simulink model "Flux_Nonsensor_pmsm"  (R2024a)
settings: Solver=FixedStepDiscrete  StartTime=0.0  StopTime=2  FixedStep=Fixed_Step_Size  RelTol=1e-3
InitFcn:
  | Flux_Nonsensor_data_new
values from neighbouring files (symbols this model uses):
  A = 1    [saddleToDuty.m]
  BandwidthCurrentPI = 1256*1.5    (= 1884)    [Flux_Nonsensor_data_new.m]
  Fixed_Step_Size = 1e-6    (= 1e-06)    [Flux_Nonsensor_data_new.m]
  Flux = 0.01837    [Flux_Nonsensor_data_new.m]
  Gamma = mpt.Parameter    [Flux_Nonsensor_data_new.m]
  Ld = 0.0001    [Flux_Nonsensor_data_new.m]
  Lq = 0.0001040    (= 0.000104)    [Flux_Nonsensor_data_new.m]
  Ls = 0.000195185    [Flux_Nonsensor_data_new.m]
  MaxVoltage = 10    [Flux_Nonsensor_data_new.m]
  pll_omega = mpt.Parameter    [Flux_Nonsensor_data_new.m]
  pll_xi = mpt.Parameter    [Flux_Nonsensor_data_new.m]
  PolePairs = 3    [Flux_Nonsensor_data_new.m]
  Rs = 0.02065    [Flux_Nonsensor_data_new.m]
  Speed_Ki = mpt.Parameter    [Flux_Nonsensor_data_new.m]
  Speed_Kp = mpt.Parameter    [Flux_Nonsensor_data_new.m]
  Speed_PI_OutputMax = 8    [Flux_Nonsensor_data_new.m]
  Speed_PI_OutputMin = -8    [Flux_Nonsensor_data_new.m]
  TsBSP = 1e-4    (= 0.0001)    [Flux_Nonsensor_data_new.m]
  TsBSP_MODEL = 2.5e-5    (= 2.5e-05)    [Flux_Nonsensor_data_new.m]
  TsFOC = 1e-4    (= 0.0001)    [Flux_Nonsensor_data_new.m]
undefined symbols (not defined in the file or in its folder): DiscIntNeverNeededParam, magnitude
libraries: slpidlib x3, mcbplantlib x1, spsDCVoltageSourceLib x1, spsGroundLib x1, autolibpmsminterior x1, spsPermanentMagnetSynchronousMachineLib x1, simulink x1, spsThreePhaseVIMeasurementLib x1, spsUniversalBridgeLib x1, sps_lib x1
settings Model: Creator=Administrator  LastModifiedBy=wanjietian
settings SolverCC: AlgebraicLoopSolver=TrustRegion
settings OptimizationCC: DefaultParameterBehavior=Inlined  UseDivisionForNetSlopeComputation=on  GainParamInheritBuiltInType=on  UseFloatMulNetSlope=on  InlineInvariantSignals=on  PassReuseOutputArgsAs=Individual arguments  ZeroExternalMemoryAtStartup=off  ZeroInternalMemoryAtStartup=off  NoFixptDivByZeroProtection=on  EfficientFloat2IntCast=on  LifeSpan=1  OptimizeBlockOrder=speed  DifferentSizesBufferReuse=on  EfficientTunableParamExpr=on
settings DebuggingCC: ParameterPrecisionLossMsg=none  ParameterTunabilityLossMsg=error  UnconnectedInputMsg=warning  UnconnectedOutputMsg=warning  UnconnectedLineMsg=warning
settings HardwareCC: ProdBitPerPointer=32  ProdBitPerSizeT=32  ProdBitPerPtrDiffT=32  ProdLargestAtomicInteger=Long  ProdLargestAtomicFloat=Double  ProdWordSize=32  ProdLongLongMode=on  ProdHWDeviceType=NXP->Cortex-M4
settings ModelReferenceCC: EnableRefExpFcnMdlSchedulingChecks=on  ModelReferenceNumInstancesAllowed=Single
settings SFSimCC: MATLABDynamicMemAlloc=off
settings RTWCC: Description=Embedded Coder  SystemTargetFile=ert.tlc  GenCodeOnly=on  TemplateMakefile=ert_default_tmf  GenerateReport=on  BuildConfiguration=Faster Runs  LaunchReport=on  GPUComputeCapability=3.5  DLArmComputeVersion=19.05
settings CodeAppCC: ForceParamTrailComments=on  IgnoreCustomStorageClasses=off  MaxIdLength=64  OperatorAnnotations=on  SimulinkDataObjDesc=on  SFDataObjDesc=on  CustomSymbolStrGlobalVar=rt$N$M  CustomSymbolStrType=$N$M  CustomSymbolStrFcn=$N$M$F  CustomSymbolStrMacro=$N$M  InsertBlockDesc=on
settings ERTTargetCC: TargetLangStandard=C99 (ISO)  GenerateSampleERTMain=on  IncludeMdlTerminateFcn=off  CombineSignalStateStructs=on  IncludeFileDelimiter=UseQuote  SupportAbsoluteTime=off  SupportComplex=off  SupportNonInlinedSFcns=on  InlinedParameterPlacement=NonHierarchical  ERTCustomFileTemplate=example_file_process.tlc  GlobalDataDefinition=InSeparateSourceFile  DataDefinitionFile=global_mcu_adc_isr.c  GlobalDataReference=InSeparateHeaderFile  DataReferenceFile=global_mcu_adc_isr.h

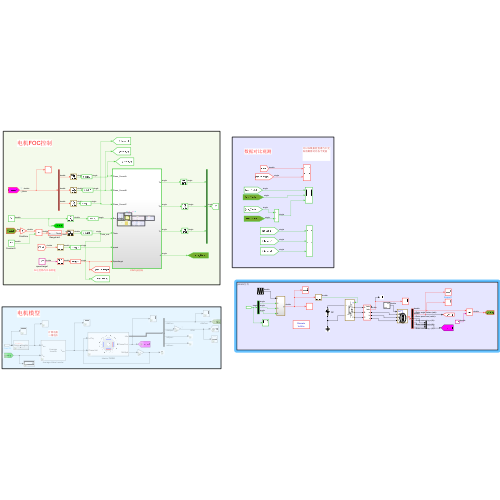
[thumbnail: Simulink's stored preview of the top-level diagram]
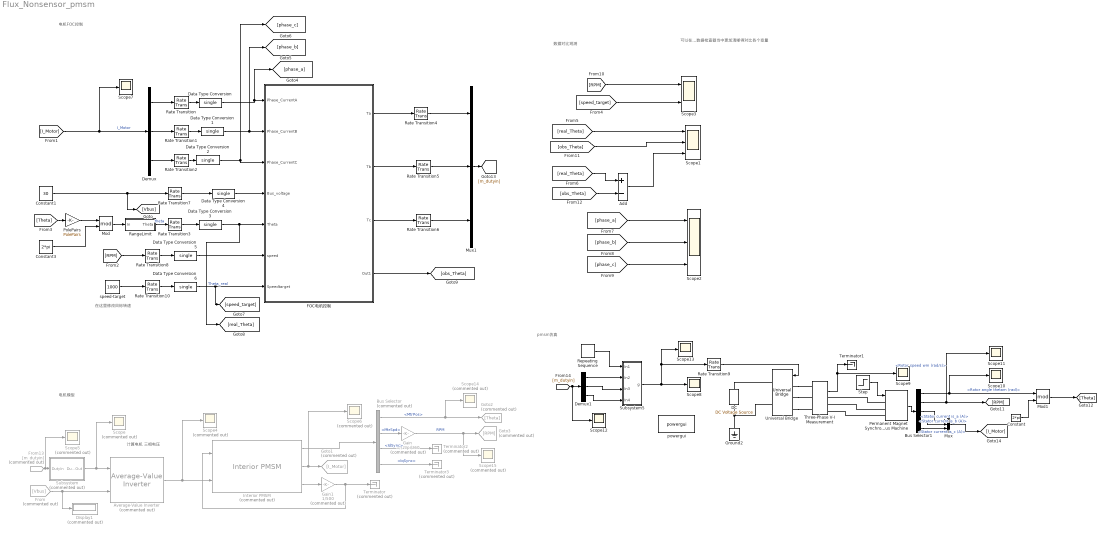
== system Flux_Nonsensor_pmsm ==
  note: pmsm仿真
  note: 可以在数据检查器当中更加清晰得对比各个变量
  note: 数据对比观测
  note: 计算电机
      | 三相电压
  note: 在这里修改目标转速
  note: 电机FOC控制
  note: 电机模型
  Add : Sum  Inputs=+-  OutDataTypeStr=single
  Average-Value Inverter : mcbplantlib/Average-Value Inverter  Commented=on
  Bus Selector : BusSelector  Commented=on  OutputSignals=MtrPos,MtrSpd,IdSync,IqSync
  Bus Selector1 : BusSelector  OutputSignals=Rotor angle thetam (rad),Rotor speed wm (rad/s),Stator current is_a (A),Stator current is_b (A),Stator current is_c (A)
  Constant : Constant  Value=2*pi
  Constant1 : Constant  Value=30  SampleTime=TsBSP
  "Constant3  " : Constant  Value=2*pi  SampleTime=TsBSP
  "DC " : spsDCVoltageSourceLib/DC Voltage Source  Amplitude=24  Measurements=Voltage
  Data Type Conversion{,1..6} (7 alike) : DataTypeConversion  OutDataTypeStr=single  SaturateOnIntegerOverflow=off  RndMeth=Floor
  Demux : Demux  Outputs=3
  Demux1 : Demux  Outputs=3
  Display1 : Display  Commented=on
  FOC电机控制 : Subsystem  TreatAsAtomicUnit=on  SystemSampleTime=TsFOC
  From : From  Commented=on  GotoTag=Vbus
  From13 : From  Commented=on  GotoTag=m_dutyin
  Gain : Gain  Commented=on  Gain=1/(2*pi)*60
  Gain1 : Gain  Commented=on  Gain=1/500
  Goto1 : Goto  Commented=on  GotoTag=I_Motor
  Goto2 : Goto  Commented=on  GotoTag=Theta
  Goto3 : Goto  Commented=on  GotoTag=RPM
  Ground2 : spsGroundLib/Ground  LConnTagsString=a
  Interior PMSM : autolibpmsminterior/Interior PMSM  Commented=on  port_config=Torque  sim_type=Discrete  Ts=TsBSP_MODEL  FilePath=interiorpmsm_motordata.m  P=PolePairs  Rs=Rs  Ldq=[Ld Lq]  KConstText=Permanent flux linkage constant (lambda_pm):  lambda_pm=Flux_MODEL  Ke=159.9771  mechanical=[2.58e-4, 8e-5, 0]  idq0=[0 0]  theta_init=0  omega_init=0  KConst=Flux_MODEL  lambda_pm_calc=Flux_MODEL  Kt=1.323  RefBlkName='autolibpmsminterior/Interior PMSM'  aMode=1
      settings: LibrarySourceBlock=autolibemachines/Interior PMSM
  Mod : Math  Operator=mod
  Mod1 : Math  Operator=mod  SignedPower=on
  Mux : Mux  Inputs=3
  Mux1 : Mux  Inputs=3
  Permanent Magnet Synchronous Machine : spsPermanentMagnetSynchronousMachineLib/Permanent Magnet Synchronous Machine  NbPhases=3  FluxDistribution=Sinusoidal  RotorType=Round  MechanicalLoad=Torque Tm  PresetModel=No  ShowDetailedParameters=on  MeasurementBus=off  Resistance=Rs  Inductance=8.5e-3  dqInductances=[8.5e-3,8.5e-3]  La=0.000395  MachineConstant=Flux linkage established by magnets (V.s)  Flux=0.1194  VoltageCst=86.6271  TorqueCst=0.7164  Flat=120  Mechanical=[0.0027 0.0004924 4 0]  PolePairs=4  InitialConditions=[0,0, 0,0]  InitialConditions5ph=[0 0 0 0 0 0]  RefAngle=90 degrees behind phase A axis (modified Park)  IterativeDiscreteModel=Trapezoidal non iterative  TsBlock=-1  TsPowergui=0
  PolePairs : Gain  Gain=PolePairs
  RangeLimit : Subsystem
  Rate Transition{,1..3,7..8,10} (7 alike) : RateTransition
  Rate Transition{4..6,9} (4 alike) : RateTransition  OutPortSampleTime=TsBSP
  Repeating Sequence : simulink/Sources/Repeating Sequence  rep_seq_t=[0 0.0001 0.0002]  rep_seq_y=[0 6000 0]
  Scope{,4..6,14..15} (6 alike) : Scope  Commented=on
  Scope1 : Scope  NumInputPorts=3
  Scope{7..13} (7 alike) : Scope
  Scope2 : Scope  NumInputPorts=3
  Scope3 : Scope  NumInputPorts=2
  Step : Step  Time=0  After=0  SampleTime=0
  Subsystem : Subsystem  Commented=on
  Subsystem5 : Subsystem
  Terminator : Terminator  Commented=on
  Terminator1 : Terminator
  Terminator2 : Terminator  Commented=on
  Terminator3 : Terminator  Commented=on
  Three-Phase V-I Measurement : spsThreePhaseVIMeasurementLib/Three-Phase V-I Measurement  VoltageMeasurement=phase-to-ground  SetLabelV=off  LabelV=Vabc  Vpu=off  VpuLL=off  CurrentMeasurement=yes  SetLabelI=off  LabelI=Iabc  Ipu=off  Pbase=100e6  Vbase=500e3  OutputType=Complex  PhasorSimulation=off  PSBequivalent=0
  Universal Bridge : spsUniversalBridgeLib/Universal Bridge  Arms=3  SnubberResistance=1e5  SnubberCapacitance=inf  Device=IGBT / Diodes  Ron=1e-3  Lon=0  ForwardVoltages="[  0  0  ]"  ForwardVoltage=0  GTOparameters=[ 10e-6 , 20e-6 ]  IGBTparameters=[ 1e-6 , 2e-6 ]  Measurements=All voltages and currents  Measurements_2=None  converterType=Rectifier
  powergui : sps_lib/powergui  Priority=1  SimulationMode=Discrete  SampleTime=Fixed_Step_Size  frequency=60  Iterations=50  frequencyindice=0  Pbase=100e6  ErrMax=1e-4  UnitsV=kV  UnitsW=MW  buscounter=0  FunctionMessages=off  echomessages=off  EnableUseOfTLC=off  CurrentSourceSwitches=off  DisableSnubberDevices=off  DisableRonSwitches=off  DisableVfSwitches=off  DisplayEquations=off  AutomaticDiscreteSolvers=off  SolverType=Tustin/Backward Euler (TBE)  Interpol=off  ExternalGateDelay=off  methode=off  Ts=100  x0status=blocks  SPID=on  SwTol=0  HookPort=off  NonlinearTolerance=1e-4  nMaxIteration=100  ContinueOnMaxIteration=off  RestoreLinks=warning  ResistiveCurrentMeasurement=off  Frange=[0:2:500]  Ylog=off  Xlog=on  ShowGrid=off  save=off  variable=ZData  structure=0  ZoomFFT=off  StartTime=0.0  cycles=1  DisplayStyle=1  fundamental=60  FreqAxis=off  MaxFrequency=1000  frequencyindicesteady=1  RmsSteady=1  display=off
  speed-target : Constant  Value=1000
  wires:
  Data Type Conversion3/1 -> [real_Theta], FOC电机控制/5(Theta)  "Theta_real"
  FOC电机控制/2(Tb) -> Rate Transition5/1
  Demux/2 -> Rate Transition1/1
  FOC电机控制/1(Ta) -> Rate Transition4/1
  [I_Motor] -> Scope7/1, Demux/1  "I_Motor"
  "Constant3  "/1 -> Mod/2
  RangeLimit/1(Theta) -> Rate Transition3/1  "theta"
  Rate Transition6/1 -> Mux1/3
  PolePairs/1 -> Mod/1
  Rate Transition5/1 -> Mux1/2
  Rate Transition3/1 -> Data Type Conversion3/1
  Data Type Conversion4/1 -> FOC电机控制/4(Bus_voltage)
  Data Type Conversion/1 -> [phase_a], FOC电机控制/1(Phase_CurrentA)
  Rate Transition7/1 -> Data Type Conversion4/1
  Rate Transition1/1 -> Data Type Conversion1/1
  Rate Transition4/1 -> Mux1/1
  Rate Transition2/1 -> Data Type Conversion2/1
  Demux/1 -> Rate Transition/1
  Demux/3 -> Rate Transition2/1
  Constant1/1 -> [Vbus], Rate Transition7/1
  FOC电机控制/3(Tc) -> Rate Transition6/1
  Rate Transition/1 -> Data Type Conversion/1
  Mod/1 -> RangeLimit/1(In)
  Data Type Conversion1/1 -> [phase_b], FOC电机控制/2(Phase_CurrentB)
  Data Type Conversion2/1 -> [phase_c], FOC电机控制/3(Phase_CurrentC)
  [Theta] -> PolePairs/1
  Bus Selector/2 -> Gain/1  "<MtrSpd>"
  Subsystem/1(DutyOut) -> Scope/1, Average-Value Inverter/1
  Bus Selector/4 -> Terminator3/1  "<IqSync>"
  Gain1/1 -> Interior PMSM/1, Terminator/1
  Bus Selector/3 -> Terminator2/1  "<IdSync>"
  Gain/1 -> Scope15/1, Goto3/1  "RPM"
  From/1 -> Display1/1, Average-Value Inverter/2
  Bus Selector/1 -> Scope14/1, Goto2/1  "<MtrPos>"
  Rate Transition8/1 -> Data Type Conversion5/1
  [RPM] -> Rate Transition8/1
  Data Type Conversion5/1 -> FOC电机控制/6(speed)
  Average-Value Inverter/1 -> Scope4/1, Interior PMSM/2
  Interior PMSM/3 -> Gain1/1
  Interior PMSM/1 -> Bus Selector/1
  speed-target/1 -> Rate Transition10/1
  Data Type Conversion6/1 -> [speed_target], FOC电机控制/7(Speedtarget)
  Rate Transition10/1 -> Data Type Conversion6/1
  [real_Theta] -> Scope1/1
  [phase_a] -> Scope2/1
  [phase_b] -> Scope2/2
  [phase_c] -> Scope2/3
  [RPM] -> Scope3/1
  [speed_target] -> Scope3/2
  FOC电机控制/4(Out1) -> [obs_Theta]
  [obs_Theta] -> Scope1/2
  [real_Theta] -> Add/1
  [obs_Theta] -> Add/2
  Add/1 -> Scope1/3
  Interior PMSM/2 -> Scope6/1, Goto1/1
  Repeating Sequence/1 -> Subsystem5/1(In1)
  Demux1/2 -> Subsystem5/3(In3)
  Demux1/1 -> Subsystem5/2(In2)
  Demux1/3 -> Subsystem5/4(In4)
  Subsystem5/1(g) -> Scope13/1, Rate Transition9/1, Scope8/1
  Rate Transition9/1 -> Universal Bridge/1
  Three-Phase V-I Measurement/2 -> Terminator1/1, Scope9/1
  Permanent Magnet Synchronous Machine/1 -> Bus Selector1/1
  Bus Selector1/1 -> Scope10/1, Mod1/1  "<Rotor angle thetam (rad)>"
  Bus Selector1/2 -> [RPM], Scope11/1  "<Rotor speed wm (rad/s)>"
  Constant/1 -> Mod1/2
  Mod1/1 -> [Theta]
  Mux1/1 -> [m_dutyin]
  From13/1 -> Scope5/1, Subsystem/1(DutyIn)
  [m_dutyin] -> Scope12/1, Demux1/1
  Step/1 -> Permanent Magnet Synchronous Machine/1
  Bus Selector1/3 -> Mux/1  "<Stator current is_a (A)>"
  Bus Selector1/4 -> Mux/2  "<Stator current is_b (A)>"
  Bus Selector1/5 -> Mux/3  "<Stator current is_c (A)>"
  Mux/1 -> [I_Motor]
  connections:
  Universal Bridge/LConn1 -- Three-Phase V-I Measurement/LConn1
  Universal Bridge/LConn2 -- Three-Phase V-I Measurement/LConn2
  Universal Bridge/LConn3 -- Three-Phase V-I Measurement/LConn3
  "DC "/RConn1 -- Universal Bridge/RConn1
  "DC "/LConn1 -- Ground2/LConn1 -- Universal Bridge/RConn2
  Permanent Magnet Synchronous Machine/LConn1 -- Three-Phase V-I Measurement/RConn1
  Permanent Magnet Synchronous Machine/LConn2 -- Three-Phase V-I Measurement/RConn2
  Permanent Magnet Synchronous Machine/LConn3 -- Three-Phase V-I Measurement/RConn3

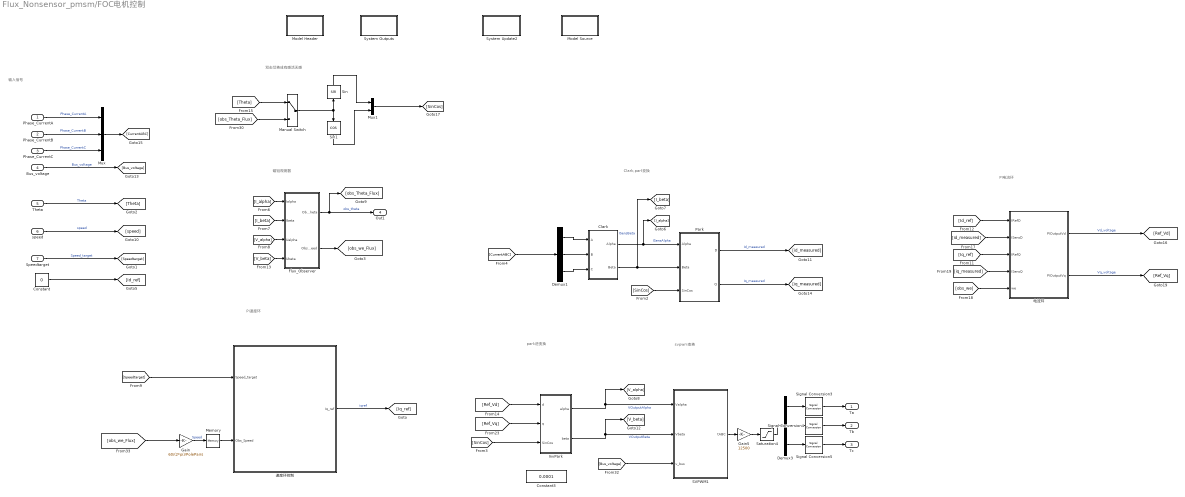
== system Flux_Nonsensor_pmsm/FOC电机控制 ==
  note: PI电流环
  note: 磁链观测器
  note: svpwm变换
  note: Clark,park变换
  note: park逆变换
  note: PI速度环
  note: 输入信号
  note: 双击切换成有感活无感
  Phase_CurrentA : Inport
  Phase_CurrentB : Inport  Port=2
  Phase_CurrentC : Inport  Port=3
  Bus_voltage : Inport  Port=4
  Theta : Inport  Port=5
  speed : Inport  Port=6
  Speedtarget : Inport  Port=7
  Clark : Subsystem  TreatAsAtomicUnit=on
      settings: RTWSystemCode=Inline  RTWFcnNameOpts=Use subsystem name
      mask Display:
      | port_label('input',1,'a','texmode','on');
      | port_label('input',2,'b','texmode','on');
      | port_label('input',3,'c','texmode','on');
      | 
      | port_label('output',1,'\alpha','texmode','on');
      | port_label('output',2,'\beta','texmode','on');
      | 
      | fprintf('Clark');
  Constant : Constant  Value=0  OutDataTypeStr=single
  Constant3 : Constant  Value=0.0001  OutDataTypeStr=single
  Demux1 : Demux  Outputs=3
  Demux3 : Demux  Outputs=3
  Flux_Observer : Subsystem
  Gain : Gain  Gain=60/(2*pi)/PolePairs
  Gain5 : Gain  Gain=12500
  InvPark : Subsystem  TreatAsAtomicUnit=on
      settings: RTWFcnNameOpts=Use subsystem name
      mask Display:
      | port_label('input',1,'d','texmode','on');
      | port_label('input',2,'q','texmode','on');
      | port_label('input',3,'\theta','texmode','on');
      | 
      | port_label('output',1,'\alpha','texmode','on');
      | port_label('output',2,'\beta','texmode','on');
      | 
      | fprintf('Inverse\nPark')
  Manual Switch : ManualSwitch
  Memory : Memory  InheritSampleTime=on
  Model Header : Subsystem  mask(Model Header){ShowInLibBrowser=0}
      mask prompts: ShowInLibBrowser "Simulink:masks:CustCodeMaskParam1_MP"
      settings: CopyFcn=cccopyfcn(gcb)  OpenFcn=ccopenfcn('Model Header')
      mask Help: eval('feval(''rtwprivate'',''rtwhelpview'',''rtw_model_header_block'')');
      mask Display: disp('Model\nHeader');
  Model Source : Subsystem  mask(Model Source){ShowInLibBrowser=0}
      mask prompts: ShowInLibBrowser "Simulink:masks:CustCodeMaskParam1_MP"
      settings: CopyFcn=cccopyfcn(gcb)  OpenFcn=ccopenfcn('Model Source')
      mask Help: eval('feval(''rtwprivate'',''rtwhelpview'',''rtw_model_source_block'')');
      mask Display: disp('Model\nSource');
  Mux : Mux  Inputs=3
  Mux1 : Mux  Inputs=2
  Park : Subsystem  TreatAsAtomicUnit=on
      settings: RTWFcnNameOpts=Use subsystem name
      mask Display:
      | port_label('input',1,'\alpha','texmode','on');
      | port_label('input',2, '\beta','texmode','on');
      | port_label('input',3, '\theta','texmode','on');
      | 
      | port_label('output',1,'d','texmode','on');
      | port_label('output',2,'q','texmode','on');
      | fprintf('Park');
  SVPWM1 : Subsystem  TreatAsAtomicUnit=on
  Saturation4 : Saturate  UpperLimit=12500  LowerLimit=0
  Signal Conversion3 : SignalConversion  OverrideOpt=off
  Signal Conversion4 : SignalConversion  OverrideOpt=off
  Signal Conversion5 : SignalConversion  OverrideOpt=off
  Sin : Trigonometry
  Sin1 : Trigonometry  Operator=cos
  System Outputs : Subsystem  mask(System Outputs){ShowInLibBrowser=0}
      mask prompts: ShowInLibBrowser "Simulink:masks:CustCodeMaskParam1_MP"
      settings: CopyFcn=cccopyfcn(gcb)  OpenFcn=ccopenfcn('System Outputs Function')
      mask Help: eval('feval(''rtwprivate'',''rtwhelpview'',''rtw_sys_outputs_block'')');
      mask Display: disp('System\nOutputs');
  System Update2 : Subsystem  mask(System Update){ShowInLibBrowser=0}
      mask prompts: ShowInLibBrowser "Simulink:masks:CustCodeMaskParam1_MP"
      settings: CopyFcn=cccopyfcn(gcb)  OpenFcn=ccopenfcn('System Update Function')
      mask Help: eval('feval(''rtwprivate'',''rtwhelpview'',''rtw_sys_update_block'')');
      mask Display: disp('System\nUpdate');
  电流环 : Subsystem  TreatAsAtomicUnit=on
  速度环控制 : Subsystem  TreatAsAtomicUnit=on
      settings: RTWSystemCode=Nonreusable function  RTWFcnNameOpts=Use subsystem name  RTWFileNameOpts=Use subsystem name  FunctionInterfaceSpec=Allow arguments (Optimized)
  Ta : Outport
  Tb : Outport  Port=2
  Tc : Outport  Port=3
  Out1 : Outport  Port=4  OutDataTypeStr=single
  wires:
  Phase_CurrentC/1 -> Mux/3  "Phase_CurrentC"
  Phase_CurrentA/1 -> Mux/1  "Phase_CurrentA"
  Phase_CurrentB/1 -> Mux/2  "Phase_CurrentB"
  Bus_voltage/1 -> [Bus_voltage]  "Bus_voltage"
  [Speedtarget] -> 速度环控制/1(Speed_target)
  Clark/2(Beta) -> [I_beta], Park/2(Beta)  "ISensBeta"
  [SinCos] -> Park/3(SinCos)
  InvPark/2(beta) -> [V_beta], SVPWM1/2(Vbeta)  "VOutputBeta"
  电流环/2(PIOutputVq) -> [Ref_Vq]  "Vq_voltage"
  电流环/1(PIOutputVd) -> [Ref_Vd]  "Vd_voltage"
  Flux_Observer/2(Obs_Speed) -> [obs_we_Flux]
  Demux1/3 -> Clark/3(C)
  [I_alpha] -> Flux_Observer/1(Ialpha)
  [V_alpha] -> Flux_Observer/3(Ualpha)
  Demux1/2 -> Clark/2(B)
  Clark/1(Alpha) -> [I_alpha], Park/1(Alpha)  "ISensAlpha"
  Demux1/1 -> Clark/1(A)
  [I_beta] -> Flux_Observer/2(Ibeta)
  [V_beta] -> Flux_Observer/4(Ubeta)
  [Id_ref] -> 电流环/1(IRefD)
  [SinCos] -> InvPark/3(SinCos)
  [Iq_ref] -> 电流环/3(IRefQ)
  [CurrentABC] -> Demux1/1
  InvPark/1(alpha) -> [V_alpha], SVPWM1/1(Valpha)  "VOutputAlpha"
  Mux/1 -> [CurrentABC]
  Theta/1 -> [Theta]  "Theta"
  speed/1 -> [speed]  "speed"
  Speedtarget/1 -> [Speedtarget]  "Speed_target"
  [obs_we_Flux] -> Gain/1
  Gain/1 -> Memory/1  "Speed"
  速度环控制/1(Iq_ref) -> [Iq_ref]  "iqref"
  Sin1/1 -> Mux1/2
  Sin/1 -> Mux1/1
  [obs_we] -> 电流环/5(we)
  Memory/1 -> 速度环控制/2(Obs_Speed)
  Flux_Observer/1(Obs_Theta) -> [obs_Theta_Flux], Out1/1  "obs_theta"
  Park/1(D) -> [id_measured]  "Id_measured"
  Park/2(Q) -> [iq_measured]  "Iq_measured"
  [id_measured] -> 电流环/2(ISensD)
  [iq_measured] -> 电流环/4(ISensQ)
  [Ref_Vd] -> InvPark/1(d)
  [Ref_Vq] -> InvPark/2(q)
  Constant/1 -> [Id_ref]
  [Theta] -> Manual Switch/1
  [obs_Theta_Flux] -> Manual Switch/2
  Manual Switch/1 -> Sin1/1, Sin/1
  Mux1/1 -> [SinCos]
  Demux3/1 -> Signal Conversion3/1
  SVPWM1/1(tABC) -> Gain5/1
  Demux3/3 -> Signal Conversion5/1
  Demux3/2 -> Signal Conversion4/1
  Saturation4/1 -> Demux3/1
  Gain5/1 -> Saturation4/1
  [Bus_voltage] -> SVPWM1/3(v_bus)
  Signal Conversion3/1 -> Ta/1
  Signal Conversion4/1 -> Tb/1
  Signal Conversion5/1 -> Tc/1

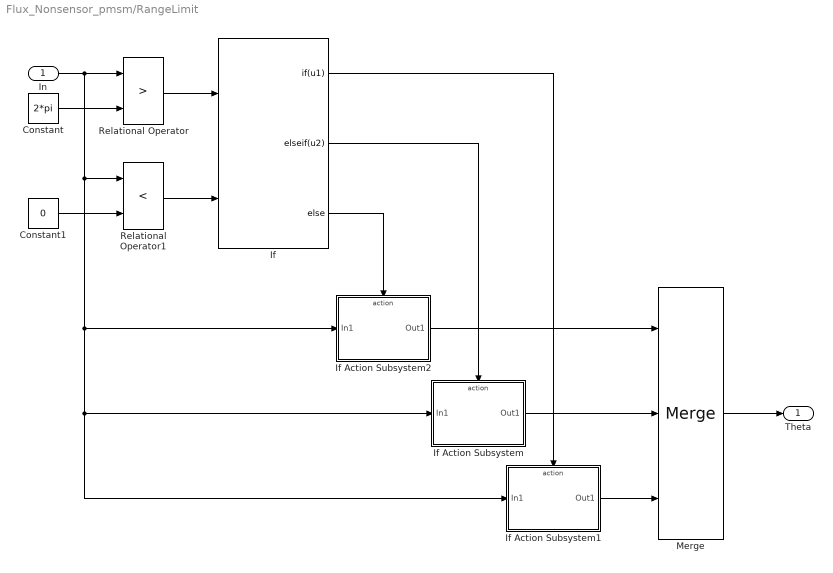
== system Flux_Nonsensor_pmsm/RangeLimit ==
  In : Inport
  Constant : Constant  Value=2*pi  OutDataTypeStr=single  SampleTime=-1
  Constant1 : Constant  Value=0  OutDataTypeStr=single  SampleTime=-1
  If : If  NumInputs=2  IfExpression=u1  ElseIfExpressions=u2
  If Action Subsystem : Subsystem  TreatAsAtomicUnit=on
  If Action Subsystem1 : Subsystem  TreatAsAtomicUnit=on
  If Action Subsystem2 : Subsystem  TreatAsAtomicUnit=on
  Merge : Merge  Inputs=3
  Relational Operator : RelationalOperator  Operator=>  OutDataTypeStr=boolean  RndMeth=Simplest  InputSameDT=off
  Relational Operator1 : RelationalOperator  Operator=<  OutDataTypeStr=boolean  RndMeth=Simplest  InputSameDT=off
  Theta : Outport
  wires:
  Relational Operator/1 -> If/1
  Constant/1 -> Relational Operator/2
  Constant1/1 -> Relational Operator1/2
  In/1 -> Relational Operator1/1, If Action Subsystem2/1(In1), If Action Subsystem1/1(In1), If Action Subsystem/1(In1), Relational Operator/1
  Relational Operator1/1 -> If/2
  Merge/1 -> Theta/1
  If/3 -> If Action Subsystem2/Action
  If/2 -> If Action Subsystem/Action
  If/1 -> If Action Subsystem1/Action
  If Action Subsystem2/1(Out1) -> Merge/1
  If Action Subsystem/1(Out1) -> Merge/2
  If Action Subsystem1/1(Out1) -> Merge/3

== system Flux_Nonsensor_pmsm/Subsystem ==
  note: 注：该模块用于将输出pwm值，将ta，tb，tc的值变成可用于与三角载波比较的值，即占空比值，用于后面计算电机三相电压
  DutyIn : Inport
  Constant : Constant  Value=0.5  SampleTime=TsBSP
  Gain : Gain  Gain=1/12500  ParamDataTypeStr=single
  Gain1 : Gain  Gain=-1
  Sum : Sum  Inputs=|+-
  Sum1 : Sum  Inputs=|++
  DutyOut : Outport
  wires:
  Sum/1 -> Gain1/1
  Constant/1 -> Sum1/2, Sum/2
  DutyIn/1 -> Gain/1
  Gain1/1 -> Sum1/1
  Sum1/1 -> DutyOut/1
  Gain/1 -> Sum/1

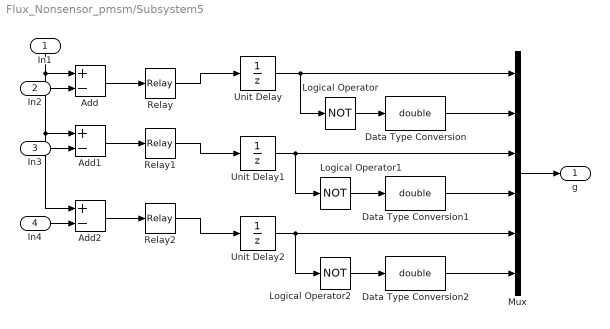
== system Flux_Nonsensor_pmsm/Subsystem5 ==
  In1 : Inport
  In2 : Inport  Port=2
  In3 : Inport  Port=3
  In4 : Inport  Port=4
  Add : Sum  Inputs=+-
  Add1 : Sum  Inputs=+-
  Add2 : Sum  Inputs=+-
  Data Type Conversion : DataTypeConversion  OutDataTypeStr=double  SaturateOnIntegerOverflow=off  RndMeth=Floor
  Data Type Conversion1 : DataTypeConversion  OutDataTypeStr=double  SaturateOnIntegerOverflow=off  RndMeth=Floor
  Data Type Conversion2 : DataTypeConversion  OutDataTypeStr=double  SaturateOnIntegerOverflow=off  RndMeth=Floor
  Logical Operator : Logic  Operator=NOT  AllPortsSameDT=off  OutDataTypeStr=boolean
  Logical Operator1 : Logic  Operator=NOT  AllPortsSameDT=off  OutDataTypeStr=boolean
  Logical Operator2 : Logic  Operator=NOT  AllPortsSameDT=off  OutDataTypeStr=boolean
  Mux : Mux  Inputs=6
  Relay : Relay  OffSwitchValue=-eps
  Relay1 : Relay  OffSwitchValue=-eps
  Relay2 : Relay  OffSwitchValue=-eps
  Unit Delay : UnitDelay  SampleTime=-1  HasFrameUpgradeWarning=on
  Unit Delay1 : UnitDelay  SampleTime=-1  HasFrameUpgradeWarning=on
  Unit Delay2 : UnitDelay  SampleTime=-1  HasFrameUpgradeWarning=on
  g : Outport  VectorParamsAs1DForOutWhenUnconnected=off
  wires:
  In4/1 -> Add2/2
  In3/1 -> Add1/2
  In2/1 -> Add/2
  Relay2/1 -> Unit Delay2/1
  Relay1/1 -> Unit Delay1/1
  Relay/1 -> Unit Delay/1
  Unit Delay2/1 -> Mux/5, Logical Operator2/1
  Unit Delay1/1 -> Mux/3, Logical Operator1/1
  Unit Delay/1 -> Logical Operator/1, Mux/1
  Mux/1 -> g/1
  Data Type Conversion/1 -> Mux/2
  Data Type Conversion1/1 -> Mux/4
  Data Type Conversion2/1 -> Mux/6
  Logical Operator2/1 -> Data Type Conversion2/1
  Logical Operator1/1 -> Data Type Conversion1/1
  Logical Operator/1 -> Data Type Conversion/1
  Add1/1 -> Relay1/1
  Add2/1 -> Relay2/1
  Add/1 -> Relay/1
  In1/1 -> Add/1, Add2/1, Add1/1

== system Flux_Nonsensor_pmsm/FOC电机控制/Clark ==
  A : Inport  OutDataTypeStr=single
  B : Inport  Port=2  OutDataTypeStr=single
  C : Inport  Port=3  OutDataTypeStr=single
  Gain : Gain  Gain=single(2/3)  OutDataTypeStr=single
  Gain1 : Gain  Gain=0.5  OutDataTypeStr=single
  Gain2 : Gain  Gain=single(sqrt(3)/3)  OutDataTypeStr=single
  Sum : Sum  Inputs=|++  OutDataTypeStr=single
  Sum1 : Sum  Inputs=|+-  OutDataTypeStr=single
  Sum2 : Sum  Inputs=+-|  OutDataTypeStr=single
  Alpha : Outport  OutDataTypeStr=single
  Beta : Outport  Port=2  OutDataTypeStr=single
  wires:
  Sum/1 -> Gain1/1
  Gain2/1 -> Beta/1
  B/1 -> Sum2/1, Sum/1
  Gain1/1 -> Sum1/2
  Gain/1 -> Alpha/1
  Sum2/1 -> Gain2/1
  C/1 -> Sum2/2, Sum/2
  A/1 -> Sum1/1
  Sum1/1 -> Gain/1

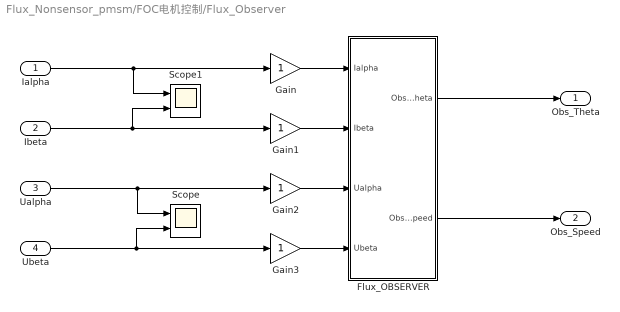
== system Flux_Nonsensor_pmsm/FOC电机控制/Flux_Observer ==
  Ialpha : Inport  OutDataTypeStr=single
  Ibeta : Inport  Port=2  OutDataTypeStr=single
  Ualpha : Inport  Port=3  OutDataTypeStr=single
  Ubeta : Inport  Port=4  OutDataTypeStr=single
  Flux_OBSERVER : Subsystem
  Gain{,1..3} (4 alike) : Gain
  Scope : Scope  NumInputPorts=2
  Scope1 : Scope  NumInputPorts=2
  Obs_Theta : Outport
  Obs_Speed : Outport  Port=2
  wires:
  Ibeta/1 -> Scope1/2, Gain1/1
  Ualpha/1 -> Scope/1, Gain2/1
  Ubeta/1 -> Scope/2, Gain3/1
  Ialpha/1 -> Scope1/1, Gain/1
  Gain/1 -> Flux_OBSERVER/1(Ialpha)
  Gain1/1 -> Flux_OBSERVER/2(Ibeta)
  Gain2/1 -> Flux_OBSERVER/3(Ualpha)
  Gain3/1 -> Flux_OBSERVER/4(Ubeta)
  Flux_OBSERVER/1(Obs_Theta) -> Obs_Theta/1
  Flux_OBSERVER/2(Obs_Speed) -> Obs_Speed/1

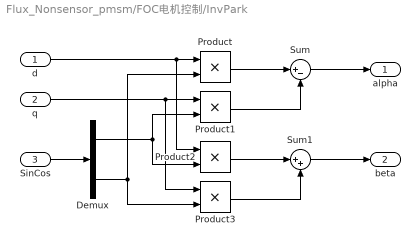
== system Flux_Nonsensor_pmsm/FOC电机控制/InvPark ==
  d : Inport  OutDataTypeStr=single
  q : Inport  Port=2  OutDataTypeStr=single
  SinCos : Inport  Port=3  OutDataTypeStr=single
  Demux : Demux  Outputs=2
  Product{,1..3} (4 alike) : Product  OutDataTypeStr=single
  Sum : Sum  Inputs=|+-  OutDataTypeStr=single
  Sum1 : Sum  Inputs=|++  OutDataTypeStr=single
  alpha : Outport  OutDataTypeStr=single
  beta : Outport  Port=2  OutDataTypeStr=single
  wires:
  Sum/1 -> alpha/1
  SinCos/1 -> Demux/1
  d/1 -> Product2/1, Product/1
  Demux/2 -> Product/2, Product3/2
  q/1 -> Product3/1, Product1/1
  Demux/1 -> Product1/2, Product2/2
  Product/1 -> Sum/1
  Product1/1 -> Sum/2
  Product2/1 -> Sum1/1
  Product3/1 -> Sum1/2
  Sum1/1 -> beta/1

== system Flux_Nonsensor_pmsm/FOC电机控制/Model Header ==

== system Flux_Nonsensor_pmsm/FOC电机控制/Model Source ==

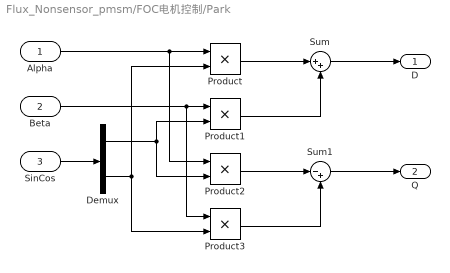
== system Flux_Nonsensor_pmsm/FOC电机控制/Park ==
  Alpha : Inport  OutDataTypeStr=single
  Beta : Inport  Port=2  OutDataTypeStr=single
  SinCos : Inport  Port=3  OutDataTypeStr=single
  Demux : Demux  Outputs=2
  Product{,1..3} (4 alike) : Product  OutDataTypeStr=single
  Sum : Sum  Inputs=|++  OutDataTypeStr=single
  Sum1 : Sum  Inputs=|-+  OutDataTypeStr=single
  D : Outport  OutDataTypeStr=single
  Q : Outport  Port=2  OutDataTypeStr=single
  wires:
  Beta/1 -> Product3/1, Product1/1
  Alpha/1 -> Product2/1, Product/1
  SinCos/1 -> Demux/1
  Demux/2 -> Product/2, Product3/2
  Demux/1 -> Product1/2, Product2/2
  Product/1 -> Sum/1
  Product1/1 -> Sum/2
  Sum/1 -> D/1
  Product2/1 -> Sum1/1
  Product3/1 -> Sum1/2
  Sum1/1 -> Q/1

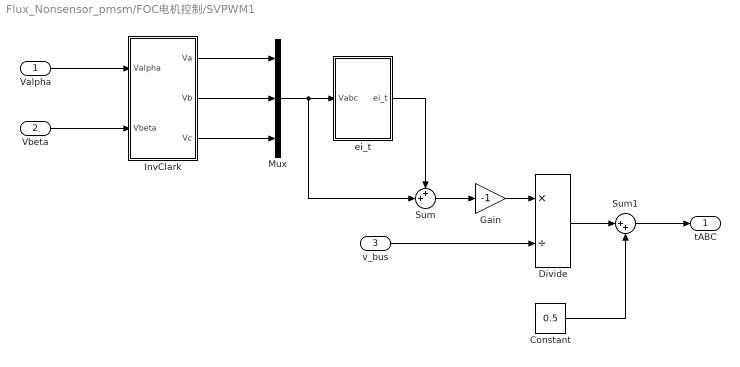
== system Flux_Nonsensor_pmsm/FOC电机控制/SVPWM1 ==
  Valpha : Inport  OutDataTypeStr=single
  Vbeta : Inport  Port=2  OutDataTypeStr=single
  v_bus : Inport  Port=3  OutDataTypeStr=single
  Constant : Constant  Value=0.5  OutDataTypeStr=single
  Divide : Product  Inputs=*/  OutDataTypeStr=single
  Gain : Gain  Gain=-1  OutDataTypeStr=single
  InvClark : Subsystem
  Mux : Mux  Inputs=3
  Sum : Sum  Inputs=++|  OutDataTypeStr=single
  Sum1 : Sum  Inputs=|++  OutDataTypeStr=single
  ei_t : Subsystem
  tABC : Outport  OutDataTypeStr=single
  wires:
  Valpha/1 -> InvClark/1(Valpha)
  Vbeta/1 -> InvClark/2(Vbeta)
  ei_t/1(ei_t) -> Sum/1
  InvClark/1(Va) -> Mux/1
  InvClark/2(Vb) -> Mux/2
  InvClark/3(Vc) -> Mux/3
  Sum/1 -> Gain/1
  Mux/1 -> Sum/2, ei_t/1(Vabc)
  Divide/1 -> Sum1/1
  Constant/1 -> Sum1/2
  v_bus/1 -> Divide/2
  Gain/1 -> Divide/1
  Sum1/1 -> tABC/1

== system Flux_Nonsensor_pmsm/FOC电机控制/System Outputs ==

== system Flux_Nonsensor_pmsm/FOC电机控制/System Update2 ==

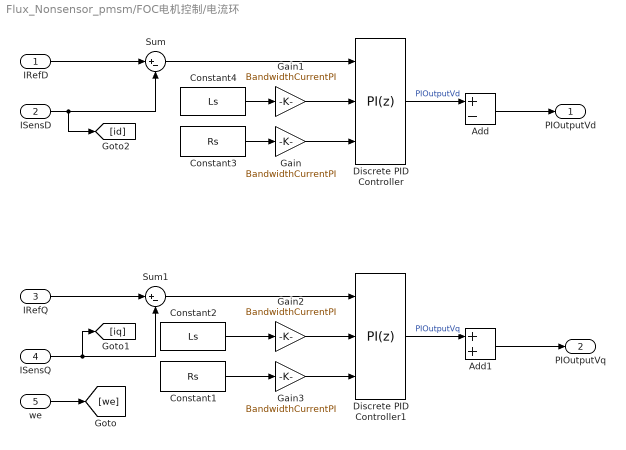
== system Flux_Nonsensor_pmsm/FOC电机控制/电流环 ==
  IRefD : Inport  OutDataTypeStr=single
  ISensD : Inport  Port=2  OutDataTypeStr=single
  IRefQ : Inport  Port=3  OutDataTypeStr=single
  ISensQ : Inport  Port=4  OutDataTypeStr=single
  we : Inport  Port=5
  Add : Sum  Inputs=+-
  Add1 : Sum
  Constant1 : Constant  Value=Rs  OutDataTypeStr=single  SampleTime=-1
  Constant2 : Constant  Value=Ls  OutDataTypeStr=single  SampleTime=-1
  Constant3 : Constant  Value=Rs  OutDataTypeStr=single  SampleTime=-1
  Constant4 : Constant  Value=Ls  OutDataTypeStr=single  SampleTime=-1
  Discrete PID Controller : slpidlib/PID Controller  Controller=PI  Form=Parallel  TimeDomain=Discrete-time  UseExternalTs=off  SampleTime=-1  IntegratorMethod=Forward Euler  FilterMethod=Forward Euler  ControllerParametersSource=external  P=1  I=1  UseKiTs=off  D=0  UseExternalDerivativeSource=off  N=100  UseFilter=off  TunerSelectOption=Transfer Function Based (PID Tuner App)  ZeroCross=off  InitialConditionSource=internal  InitialConditionForIntegrator=0  InitialConditionForFilter=0  DifferentiatorICPrevScaledInput=0  ExternalReset=none  TrackingMode=off  Kt=1  LimitOutput=on  SatLimitsSource=internal  UpperSaturationLimit=MaxVoltage*2  LowerSaturationLimit=-MaxVoltage*2  LinearizeAsGain=off  AntiWindupMode=clamping  Kb=1  LimitIntegrator=off  UpperIntegratorSaturationLimit=inf  LowerIntegratorSaturationLimit=-inf  POutMin=[]  POutMax=[]  IOutMin=[]  IOutMax=[]  DOutMin=[]  DOutMax=[]  NOutMin=[]  NOutMax=[]  SumOutMin=[]  SumOutMax=[]  SaturationOutDataTypeStr=Inherit: Inherit via back propagation  SaturationOutMin=[]  SaturationOutMax=[]  PParamMin=[]  PParamMax=[]  IParamMin=[]  IParamMax=[]  DParamMin=[]  DParamMax=[]  NParamMin=[]  NParamMax=[]  KbParamMin=[]  KbParamMax=[]  KtParamMin=[]  KtParamMax=[]  KbOutMin=[]  KbOutMax=[]  KtOutMin=[]  KtOutMax=[]  IntegratorOutMin=[]  IntegratorOutMax=[]  FilterOutMin=[]  FilterOutMax=[]  SumI1OutMin=[]  SumI1OutMax=[]  SumI2OutMin=[]  SumI2OutMax=[]  SumI3OutMin=[]  SumI3OutMax=[]  SumI4OutMin=[]  SumI4OutMax=[]  SumDOutMin=[]  SumDOutMax=[]  DifferentiatorOutMin=[]  DifferentiatorOutMax=[]  FilterDiffOutCoefMin=[]  FilterDiffOutCoefMax=[]  ReciprocalOutMin=[]  ReciprocalOutMax=[]  SumDenOutMin=[]  SumDenOutMax=[]  SumNumOutMin=[]  SumNumOutMax=[]  DivideOutMin=[]  DivideOutMax=[]  UdiffTsProdOutMin=[]  UdiffTsProdOutMax=[]  NTsProdOutMin=[]  NTsProdOutMax=[]  UintegralTsProdOutMin=[]  UintegralTsProdOutMax=[]  UngainTsProdOutMin=[]  UngainTsProdOutMax=[]  ClampingZeroOutDataTypeStr=Inherit: Inherit via back propagation  ClampingZeroOutMin=[]  ClampingZeroOutMax=[]  FilterDenConstantOutDataTypeStr=Inherit: Inherit via back propagation  FilterDenConstantOutMin=[]  FilterDenConstantOutMax=[]  PCopyOutDataTypeStr=Inherit: Inherit via back propagation  PCopyOutMin=[]  PCopyOutMax=[]  NCopyOutDataTypeStr=Inherit: Inherit via back propagation  NCopyOutMin=[]  NCopyOutMax=[]  IntegratorContinuousStateAttributes=''  IntegratorStateMustResolveToSignalObject=off  IntegratorRTWStateStorageClass=Auto  FilterContinuousStateAttributes=''  FilterStateMustResolveToSignalObject=off  FilterRTWStateStorageClass=Auto  ParallelPVariant=ExternalParameters  IdealPVariant=Disabled  IVariant=ExternalParameters  DVariant=Disabled  IntegratorVariant=Discrete  SatVariant=Enabled  AWVariant=DiscClampingParallel  PCopyVariant=Disabled  TRVariant=Disabled  FdbkBlocksVariant=Forward  IdealPFdbkVariant=Disabled  SatFdbkVariant=Disabled  DerivativeFilterVariant=Disabled  NVariant=Disabled  NCopyVariant=Disabled_SignalSpec  FilterICVariant=Disabled  IntegratorICVariant=InternalICs  ExternalResetVariant=Disabled  TRSumVariant=Passthrough  SumFdbkVariant=Disabled  SumVariant=Sum_PI  TsampFilterVariant=InternalTs  TsampNgainVariant=Passthrough  TsampIntegralVariant=Disabled_SignalSpec  ExternalSaturationOutDataTypeStr=Inherit: Same as second input  DerivativeSourceVariant=Disabled
  Discrete PID Controller1 : slpidlib/PID Controller  Controller=PI  Form=Parallel  TimeDomain=Discrete-time  UseExternalTs=off  SampleTime=-1  IntegratorMethod=Forward Euler  FilterMethod=Forward Euler  ControllerParametersSource=external  P=1  I=1  UseKiTs=off  D=0  UseExternalDerivativeSource=off  N=100  UseFilter=off  TunerSelectOption=Transfer Function Based (PID Tuner App)  ZeroCross=off  InitialConditionSource=internal  InitialConditionForIntegrator=0  InitialConditionForFilter=0  DifferentiatorICPrevScaledInput=0  ExternalReset=none  TrackingMode=off  Kt=1  LimitOutput=on  SatLimitsSource=internal  UpperSaturationLimit=MaxVoltage*2  LowerSaturationLimit=-MaxVoltage*2  LinearizeAsGain=off  AntiWindupMode=clamping  Kb=1  LimitIntegrator=off  UpperIntegratorSaturationLimit=inf  LowerIntegratorSaturationLimit=-inf  POutMin=[]  POutMax=[]  IOutMin=[]  IOutMax=[]  DOutMin=[]  DOutMax=[]  NOutMin=[]  NOutMax=[]  SumOutMin=[]  SumOutMax=[]  SaturationOutDataTypeStr=Inherit: Inherit via back propagation  SaturationOutMin=[]  SaturationOutMax=[]  PParamMin=[]  PParamMax=[]  IParamMin=[]  IParamMax=[]  DParamMin=[]  DParamMax=[]  NParamMin=[]  NParamMax=[]  KbParamMin=[]  KbParamMax=[]  KtParamMin=[]  KtParamMax=[]  KbOutMin=[]  KbOutMax=[]  KtOutMin=[]  KtOutMax=[]  IntegratorOutMin=[]  IntegratorOutMax=[]  FilterOutMin=[]  FilterOutMax=[]  SumI1OutMin=[]  SumI1OutMax=[]  SumI2OutMin=[]  SumI2OutMax=[]  SumI3OutMin=[]  SumI3OutMax=[]  SumI4OutMin=[]  SumI4OutMax=[]  SumDOutMin=[]  SumDOutMax=[]  DifferentiatorOutMin=[]  DifferentiatorOutMax=[]  FilterDiffOutCoefMin=[]  FilterDiffOutCoefMax=[]  ReciprocalOutMin=[]  ReciprocalOutMax=[]  SumDenOutMin=[]  SumDenOutMax=[]  SumNumOutMin=[]  SumNumOutMax=[]  DivideOutMin=[]  DivideOutMax=[]  UdiffTsProdOutMin=[]  UdiffTsProdOutMax=[]  NTsProdOutMin=[]  NTsProdOutMax=[]  UintegralTsProdOutMin=[]  UintegralTsProdOutMax=[]  UngainTsProdOutMin=[]  UngainTsProdOutMax=[]  ClampingZeroOutDataTypeStr=Inherit: Inherit via back propagation  ClampingZeroOutMin=[]  ClampingZeroOutMax=[]  FilterDenConstantOutDataTypeStr=Inherit: Inherit via back propagation  FilterDenConstantOutMin=[]  FilterDenConstantOutMax=[]  PCopyOutDataTypeStr=Inherit: Inherit via back propagation  PCopyOutMin=[]  PCopyOutMax=[]  NCopyOutDataTypeStr=Inherit: Inherit via back propagation  NCopyOutMin=[]  NCopyOutMax=[]  IntegratorContinuousStateAttributes=''  IntegratorStateMustResolveToSignalObject=off  IntegratorRTWStateStorageClass=Auto  FilterContinuousStateAttributes=''  FilterStateMustResolveToSignalObject=off  FilterRTWStateStorageClass=Auto  ParallelPVariant=ExternalParameters  IdealPVariant=Disabled  IVariant=ExternalParameters  DVariant=Disabled  IntegratorVariant=Discrete  SatVariant=Enabled  AWVariant=DiscClampingParallel  PCopyVariant=Disabled  TRVariant=Disabled  FdbkBlocksVariant=Forward  IdealPFdbkVariant=Disabled  SatFdbkVariant=Disabled  DerivativeFilterVariant=Disabled  NVariant=Disabled  NCopyVariant=Disabled_SignalSpec  FilterICVariant=Disabled  IntegratorICVariant=InternalICs  ExternalResetVariant=Disabled  TRSumVariant=Passthrough  SumFdbkVariant=Disabled  SumVariant=Sum_PI  TsampFilterVariant=InternalTs  TsampNgainVariant=Passthrough  TsampIntegralVariant=Disabled_SignalSpec  ExternalSaturationOutDataTypeStr=Inherit: Same as second input  DerivativeSourceVariant=Disabled
  Gain{,1..3} (4 alike) : Gain  Gain=BandwidthCurrentPI
  Sum : Sum  Inputs=|+-  OutDataTypeStr=single
  Sum1 : Sum  Inputs=|+-  OutDataTypeStr=single
  PIOutputVd : Outport  OutDataTypeStr=single
  PIOutputVq : Outport  Port=2  OutDataTypeStr=single
  wires:
  IRefD/1 -> Sum/1
  Sum/1 -> Discrete PID Controller/1
  Constant4/1 -> Gain1/1
  Constant3/1 -> Gain/1
  IRefQ/1 -> Sum1/1
  Constant2/1 -> Gain2/1
  Sum1/1 -> Discrete PID Controller1/1
  ISensQ/1 -> [iq], Sum1/2
  Constant1/1 -> Gain3/1
  Gain/1 -> Discrete PID Controller/3
  Gain1/1 -> Discrete PID Controller/2
  Gain2/1 -> Discrete PID Controller1/2
  Gain3/1 -> Discrete PID Controller1/3
  Discrete PID Controller/1 -> Add/1  "PIOutputVd"
  we/1 -> [we]
  Add/1 -> PIOutputVd/1
  Discrete PID Controller1/1 -> Add1/1  "PIOutputVq"
  Add1/1 -> PIOutputVq/1
  ISensD/1 -> Sum/2, [id]

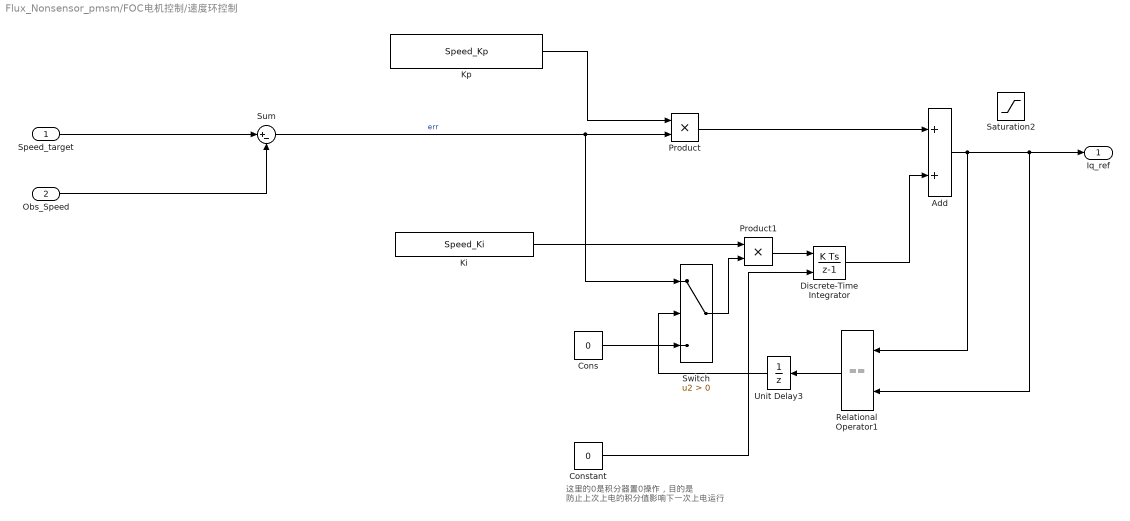
== system Flux_Nonsensor_pmsm/FOC电机控制/速度环控制 ==
  note: 这里的0是积分器置0操作，目的是
      | 防止上次上电的积分值影响下一次上电运行
  Speed_target : Inport
  Obs_Speed : Inport  Port=2  OutMin=0  OutMax=2*pi
  Add : Sum
  Cons : Constant  Value=0  OutDataTypeStr=single
  Constant : Constant  Value=0
  Discrete-Time Integrator : DiscreteIntegrator  ExternalReset=level  SampleTime=-1  ICPrevOutput=DiscIntNeverNeededParam  ICPrevScaledInput=DiscIntNeverNeededParam
  Ki : Constant  Value=Speed_Ki  OutDataTypeStr=single
  Kp : Constant  Value=Speed_Kp  OutDataTypeStr=single
  Product : Product
  Product1 : Product
  Relational Operator1 : RelationalOperator  Operator===  OutDataTypeStr=boolean  RndMeth=Simplest  InputSameDT=off
  Saturation2 : Saturate  UpperLimit=Speed_PI_OutputMax  LowerLimit=Speed_PI_OutputMin
  Sum : Sum  Inputs=|+-
  Switch : Switch  Criteria=u2 > Threshold  SaturateOnIntegerOverflow=off  InputSameDT=off
  Unit Delay3 : UnitDelay  SampleTime=-1  HasFrameUpgradeWarning=on
  Iq_ref : Outport  VectorParamsAs1DForOutWhenUnconnected=off
  wires:
  Add/1 -> Iq_ref/1, Relational Operator1/2, Relational Operator1/1
  Speed_target/1 -> Sum/1
  Obs_Speed/1 -> Sum/2
  Discrete-Time Integrator/1 -> Add/2
  Kp/1 -> Product/1
  Ki/1 -> Product1/1
  Unit Delay3/1 -> Switch/2
  Relational Operator1/1 -> Unit Delay3/1
  Switch/1 -> Product1/2
  Cons/1 -> Switch/3
  Product1/1 -> Discrete-Time Integrator/1
  Product/1 -> Add/1
  Sum/1 -> Product/2, Switch/1  "err"
  Constant/1 -> Discrete-Time Integrator/2

== system Flux_Nonsensor_pmsm/RangeLimit/If Action Subsystem ==
  In1 : Inport
  Action Port : ActionPort  ActionPortLabel=elseif(u2)
  Constant : Constant  Value=2*pi  OutDataTypeStr=single  SampleTime=-1
  Sum : Sum  Inputs=|++
  Out1 : Outport
  wires:
  In1/1 -> Sum/1
  Constant/1 -> Sum/2
  Sum/1 -> Out1/1

== system Flux_Nonsensor_pmsm/RangeLimit/If Action Subsystem1 ==
  In1 : Inport
  Action Port : ActionPort  ActionPortLabel=if(u1)
  Constant : Constant  Value=2*pi  OutDataTypeStr=single  SampleTime=-1
  Sum : Sum  Inputs=|+-
  Out1 : Outport
  wires:
  In1/1 -> Sum/1
  Constant/1 -> Sum/2
  Sum/1 -> Out1/1

== system Flux_Nonsensor_pmsm/RangeLimit/If Action Subsystem2 ==
  In1 : Inport
  Action Port : ActionPort  ActionPortLabel=else
  Out1 : Outport
  wires:
  In1/1 -> Out1/1

== system Flux_Nonsensor_pmsm/FOC电机控制/Flux_Observer/Flux_OBSERVER ==
  note: 非线性磁链观测
  note: PLL锁相环
  Ialpha : Inport  OutDataTypeStr=single
  Ibeta : Inport  Port=2  OutDataTypeStr=single
  Ualpha : Inport  Port=3  OutDataTypeStr=single
  Ubeta : Inport  Port=4  OutDataTypeStr=single
  Cacl_Flux : Subsystem
  PLL : Subsystem
  Obs_Theta : Outport
  Obs_Speed : Outport  Port=2
  wires:
  Ibeta/1 -> Cacl_Flux/4(Ibeta)
  Ialpha/1 -> Cacl_Flux/3(Ialpha)
  Ualpha/1 -> Cacl_Flux/1(Ualpha)
  Ubeta/1 -> Cacl_Flux/2(Ubeta)
  PLL/1(Obs_Theta) -> Obs_Theta/1  "Obs_Theta"
  Cacl_Flux/2(Flux_beta) -> PLL/2(Flux_beta)
  Cacl_Flux/1(Flux_alpha) -> PLL/1(Flux_alpha)
  PLL/2(Obs_we) -> Obs_Speed/1

== system Flux_Nonsensor_pmsm/FOC电机控制/SVPWM1/InvClark ==
  Valpha : Inport  OutDataTypeStr=single
  Vbeta : Inport  Port=2  OutDataTypeStr=single
  Gain : Gain  Gain=-1/2  OutDataTypeStr=single
  Gain1 : Gain  Gain=sqrt(3)/2  OutDataTypeStr=single
  Sum : Sum  Inputs=|++  OutDataTypeStr=single
  Sum1 : Sum  Inputs=-+|  OutDataTypeStr=single
  Va : Outport  OutDataTypeStr=single
  Vb : Outport  Port=2  OutDataTypeStr=single
  Vc : Outport  Port=3  OutDataTypeStr=single
  wires:
  Valpha/1 -> Gain/1, Va/1
  Vbeta/1 -> Gain1/1
  Gain/1 -> Sum1/2, Sum/1
  Sum/1 -> Vb/1
  Gain1/1 -> Sum/2, Sum1/1
  Sum1/1 -> Vc/1

== system Flux_Nonsensor_pmsm/FOC电机控制/SVPWM1/ei_t ==
  Vabc : Inport  OutDataTypeStr=single
  Demux : Demux  Outputs=3
  Gain : Gain  Gain=-1/2  OutDataTypeStr=single
  Min : MinMax  Inputs=3  OutDataTypeStr=single
  Min1 : MinMax  Function=max  Inputs=3  OutDataTypeStr=single
  Sum : Sum  Inputs=|++  OutDataTypeStr=single
  ei_t : Outport  OutDataTypeStr=single
  wires:
  Min/1 -> Sum/1
  Sum/1 -> Gain/1
  Min1/1 -> Sum/2
  Gain/1 -> ei_t/1
  Vabc/1 -> Demux/1
  Demux/1 -> Min1/1, Min/1
  Demux/2 -> Min/2, Min1/2
  Demux/3 -> Min1/3, Min/3

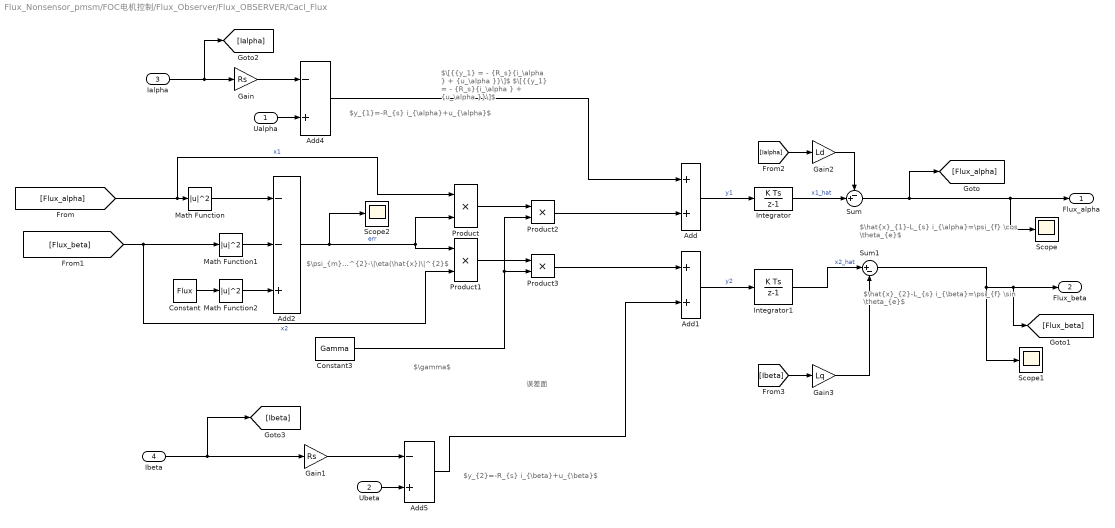
== system Flux_Nonsensor_pmsm/FOC电机控制/Flux_Observer/Flux_OBSERVER/Cacl_Flux ==
  note: 误差面
  note: $\gamma$
  note: $\psi_{m}^{2}-\|\eta(\hat{x})\|^{2}$
  note: $\hat{x}_{1}-L_{s} i_{\alpha}=\psi_{f} \cos \theta_{e}$
  note: $y_{1}=-R_{s} i_{\alpha}+u_{\alpha}$
  note: $\[{{y_1} = - {R_s}{i_\alpha } + {u_\alpha }}\]$ $\[{{y_1} = - {R_s}{i_\alpha } + {u_\alpha }}\]$
  note: $\hat{x}_{2}-L_{s} i_{\beta}=\psi_{f} \sin \theta_{e}$
  note: $y_{2}=-R_{s} i_{\beta}+u_{\beta}$
  Ualpha : Inport  OutDataTypeStr=single
  Ubeta : Inport  Port=2  OutDataTypeStr=single
  Ialpha : Inport  Port=3  OutDataTypeStr=single
  Ibeta : Inport  Port=4  OutDataTypeStr=single
  Add : Sum  OutDataTypeStr=single
  Add1 : Sum  OutDataTypeStr=single
  Add2 : Sum  Inputs=--+  OutDataTypeStr=single
  Add4 : Sum  Inputs=-+  OutDataTypeStr=single
  Add5 : Sum  Inputs=-+  OutDataTypeStr=single
  Constant : Constant  Value=Flux  OutDataTypeStr=single
  Constant3 : Constant  Value=Gamma  OutDataTypeStr=single
  Gain : Gain  Gain=Rs
  Gain1 : Gain  Gain=Rs
  Gain2 : Gain  Gain=Ld  OutDataTypeStr=single
  Gain3 : Gain  Gain=Lq  OutDataTypeStr=single
  Integrator : DiscreteIntegrator  SampleTime=-1  OutDataTypeStr=single  ICPrevOutput=DiscIntNeverNeededParam  ICPrevScaledInput=DiscIntNeverNeededParam  mask(DiscretizedDiscreteIntegrator){}
      mask init:
      | %zoh
  Integrator1 : DiscreteIntegrator  SampleTime=-1  OutDataTypeStr=single  ICPrevOutput=DiscIntNeverNeededParam  ICPrevScaledInput=DiscIntNeverNeededParam  mask(DiscretizedDiscreteIntegrator){}
      mask init:
      | %zoh
  Math Function : Math  Operator=magnitude^2  OutDataTypeStr=single
  Math Function1 : Math  Operator=magnitude^2  OutDataTypeStr=single
  Math Function2 : Math  Operator=magnitude^2  OutDataTypeStr=single
  Product{,1..3} (4 alike) : Product  OutDataTypeStr=single
  Scope : Scope
  Scope1 : Scope
  Scope2 : Scope
  Sum : Sum  Inputs=-+|  OutDataTypeStr=single
  Sum1 : Sum  Inputs=|+-  OutDataTypeStr=single
  Flux_alpha : Outport  OutDataTypeStr=single
  Flux_beta : Outport  Port=2  OutDataTypeStr=single
  wires:
  Add4/1 -> Add/1
  Product3/1 -> Add1/1
  Product1/1 -> Product3/1
  Product/1 -> Product2/1
  Product2/1 -> Add/2
  Add/1 -> Integrator/1  "y1"
  Add1/1 -> Integrator1/1  "y2"
  Add5/1 -> Add1/2
  Math Function1/1 -> Add2/2
  Math Function/1 -> Add2/1
  Add2/1 -> Scope2/1, Product1/1, Product/2  "err"
  Constant/1 -> Math Function2/1
  Math Function2/1 -> Add2/3
  [Flux_beta] -> Product1/2, Math Function1/1  "x2"
  Gain3/1 -> Sum1/2
  Integrator1/1 -> Sum1/1  "x2_hat"
  Integrator/1 -> Sum/2  "x1_hat"
  Gain2/1 -> Sum/1
  Ualpha/1 -> Add4/2
  Gain/1 -> Add4/1
  Ubeta/1 -> Add5/2
  Gain1/1 -> Add5/1
  Ibeta/1 -> [Ibeta], Gain1/1
  Ialpha/1 -> [Ialpha], Gain/1
  [Ialpha] -> Gain2/1
  [Ibeta] -> Gain3/1
  Constant3/1 -> Product2/2, Product3/2
  [Flux_alpha] -> Product/1, Math Function/1  "x1"
  Sum/1 -> Scope/1, Flux_alpha/1, [Flux_alpha]
  Sum1/1 -> Flux_beta/1, [Flux_beta], Scope1/1

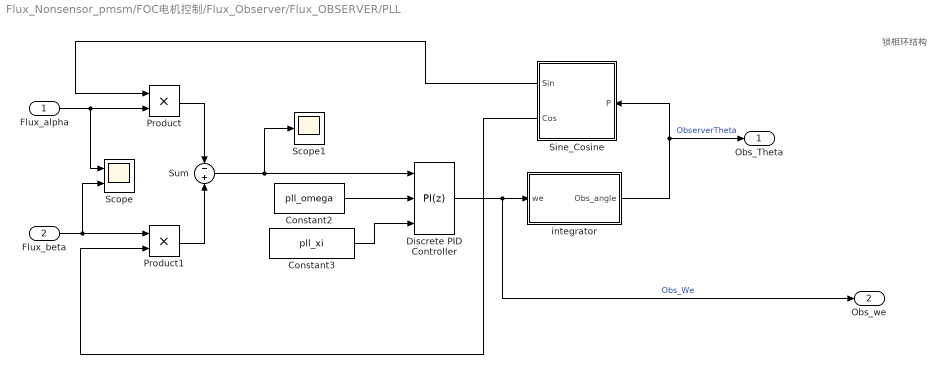
== system Flux_Nonsensor_pmsm/FOC电机控制/Flux_Observer/Flux_OBSERVER/PLL ==
  note: 锁相环结构
  Flux_alpha : Inport  OutDataTypeStr=single
  Flux_beta : Inport  Port=2  OutDataTypeStr=single
  Constant2 : Constant  Value=pll_omega  OutDataTypeStr=single
  Constant3 : Constant  Value=pll_xi  OutDataTypeStr=single
  Discrete PID Controller : slpidlib/PID Controller  Controller=PI  Form=Parallel  TimeDomain=Discrete-time  UseExternalTs=off  SampleTime=-1  IntegratorMethod=Forward Euler  FilterMethod=Forward Euler  ControllerParametersSource=external  P=2*0.707*1650  I=1650*1650  UseKiTs=off  D=0  UseExternalDerivativeSource=off  N=100  UseFilter=on  TunerSelectOption=Transfer Function Based (PID Tuner App)  ZeroCross=off  InitialConditionSource=internal  InitialConditionForIntegrator=0  InitialConditionForFilter=0  DifferentiatorICPrevScaledInput=0  ExternalReset=none  TrackingMode=off  Kt=1  LimitOutput=on  SatLimitsSource=internal  UpperSaturationLimit=3000*2*pi*PolePairs/60  LowerSaturationLimit=-3000*2*pi*PolePairs/60  LinearizeAsGain=off  AntiWindupMode=clamping  Kb=1  LimitIntegrator=off  UpperIntegratorSaturationLimit=inf  LowerIntegratorSaturationLimit=-inf  POutMin=[]  POutMax=[]  IOutMin=[]  IOutMax=[]  DOutMin=[]  DOutMax=[]  NOutMin=[]  NOutMax=[]  SumOutMin=[]  SumOutMax=[]  SaturationOutMin=[]  SaturationOutMax=[]  PParamMin=[]  PParamMax=[]  IParamMin=[]  IParamMax=[]  DParamMin=[]  DParamMax=[]  NParamMin=[]  NParamMax=[]  KbParamMin=[]  KbParamMax=[]  KtParamMin=[]  KtParamMax=[]  KbOutMin=[]  KbOutMax=[]  KtOutMin=[]  KtOutMax=[]  IntegratorOutMin=[]  IntegratorOutMax=[]  FilterOutMin=[]  FilterOutMax=[]  SumI1OutMin=[]  SumI1OutMax=[]  SumI2OutMin=[]  SumI2OutMax=[]  SumI3OutMin=[]  SumI3OutMax=[]  SumI4OutMin=[]  SumI4OutMax=[]  SumDOutMin=[]  SumDOutMax=[]  DifferentiatorOutMin=[]  DifferentiatorOutMax=[]  FilterDiffOutCoefMin=[]  FilterDiffOutCoefMax=[]  ReciprocalOutMin=[]  ReciprocalOutMax=[]  SumDenOutMin=[]  SumDenOutMax=[]  SumNumOutMin=[]  SumNumOutMax=[]  DivideOutMin=[]  DivideOutMax=[]  UdiffTsProdOutMin=[]  UdiffTsProdOutMax=[]  NTsProdOutMin=[]  NTsProdOutMax=[]  UintegralTsProdOutMin=[]  UintegralTsProdOutMax=[]  UngainTsProdOutMin=[]  UngainTsProdOutMax=[]  ClampingZeroOutDataTypeStr=Inherit: Inherit via back propagation  ClampingZeroOutMin=[]  ClampingZeroOutMax=[]  FilterDenConstantOutDataTypeStr=Inherit: Inherit via back propagation  FilterDenConstantOutMin=[]  FilterDenConstantOutMax=[]  PCopyOutDataTypeStr=Inherit: Inherit via back propagation  PCopyOutMin=[]  PCopyOutMax=[]  NCopyOutDataTypeStr=Inherit: Inherit via back propagation  NCopyOutMin=[]  NCopyOutMax=[]  IntegratorContinuousStateAttributes=''  IntegratorStateMustResolveToSignalObject=off  IntegratorRTWStateStorageClass=Auto  FilterContinuousStateAttributes=''  FilterStateMustResolveToSignalObject=off  FilterRTWStateStorageClass=Auto  ParallelPVariant=ExternalParameters  IdealPVariant=Disabled  IVariant=ExternalParameters  DVariant=Disabled  IntegratorVariant=Discrete  SatVariant=Enabled  AWVariant=DiscClampingParallel  PCopyVariant=Disabled  TRVariant=Disabled  FdbkBlocksVariant=Forward  IdealPFdbkVariant=Disabled  SatFdbkVariant=Disabled  DerivativeFilterVariant=Disabled  NVariant=Disabled  NCopyVariant=Disabled_SignalSpec  FilterICVariant=Disabled  IntegratorICVariant=InternalICs  ExternalResetVariant=Disabled  TRSumVariant=Passthrough  SumFdbkVariant=Disabled  SumVariant=Sum_PI  TsampFilterVariant=InternalTs  TsampNgainVariant=Passthrough  TsampIntegralVariant=Disabled_SignalSpec  ExternalSaturationOutDataTypeStr=Inherit: Same as second input  DerivativeSourceVariant=Disabled
  Product : Product  OutDataTypeStr=single
  Product1 : Product  OutDataTypeStr=single
  Scope : Scope  NumInputPorts=2
  Scope1 : Scope
  Sine_Cosine : Subsystem  TreatAsAtomicUnit=on
      settings: RTWSystemCode=Nonreusable function  RTWFcnNameOpts=Use subsystem name
  Sum : Sum  Inputs=-|+  OutDataTypeStr=single
  integrator : Subsystem
  Obs_Theta : Outport  OutDataTypeStr=single
  Obs_we : Outport  Port=2  OutDataTypeStr=single
  wires:
  Product/1 -> Sum/1
  Product1/1 -> Sum/2
  Sum/1 -> Scope1/1, Discrete PID Controller/1
  Sine_Cosine/2(Cos) -> Product1/2
  Sine_Cosine/1(Sin) -> Product/1
  integrator/1(Obs_angle) -> Obs_Theta/1, Sine_Cosine/1(P)  "ObserverTheta"
  Flux_alpha/1 -> Scope/1, Product/2
  Flux_beta/1 -> Scope/2, Product1/1
  Discrete PID Controller/1 -> Obs_we/1, integrator/1(we)  "Obs_We"
  Constant3/1 -> Discrete PID Controller/3
  Constant2/1 -> Discrete PID Controller/2

== system Flux_Nonsensor_pmsm/FOC电机控制/Flux_Observer/Flux_OBSERVER/PLL/Sine_Cosine ==
  note: Sine Cosine Coefficients
  P : Inport  OutDataTypeStr=single
  Cos1 : Trigonometry  Operator=cos
  Saturation : Saturate  UpperLimit=2*pi-0.001  LowerLimit=0+0.001  OutDataTypeStr=single
  Scope : Scope  NumInputPorts=2
  Sin1 : Trigonometry
  Sin : Outport  VectorParamsAs1DForOutWhenUnconnected=off
  Cos : Outport  Port=2  VectorParamsAs1DForOutWhenUnconnected=off
  wires:
  P/1 -> Saturation/1  "position"
  Sin1/1 -> Scope/1, Sin/1
  Cos1/1 -> Scope/2, Cos/1
  Saturation/1 -> Cos1/1, Sin1/1

== system Flux_Nonsensor_pmsm/FOC电机控制/Flux_Observer/Flux_OBSERVER/PLL/integrator ==
  we : Inport  OutDataTypeStr=single
  Angle_Limit : Subsystem
  Sum1 : Sum  Inputs=|++  OutDataTypeStr=single
  Ts : Gain  Gain=TsFOC  OutDataTypeStr=single
  Unit Delay : UnitDelay  SampleTime=-1  HasFrameUpgradeWarning=on
  Obs_angle : Outport  OutDataTypeStr=single
  wires:
  we/1 -> Ts/1
  Ts/1 -> Sum1/1
  Sum1/1 -> Angle_Limit/1(Angle_input)
  Unit Delay/1 -> Obs_angle/1, Sum1/2
  Angle_Limit/1(Angle_output) -> Unit Delay/1

== system Flux_Nonsensor_pmsm/FOC电机控制/Flux_Observer/Flux_OBSERVER/PLL/integrator/Angle_Limit ==
  Angle_input : Inport
  If Action Subsystem1 : Subsystem  TreatAsAtomicUnit=on
  If Action Subsystem2 : Subsystem  TreatAsAtomicUnit=on
  If Action Subsystem3 : Subsystem  TreatAsAtomicUnit=on
  If1 : If  IfExpression=u1 > 6.283185307  ElseIfExpressions=u1<0
  Merge1 : Merge  Inputs=3
  Angle_output : Outport
  wires:
  If1/2 -> If Action Subsystem3/Action
  If1/1 -> If Action Subsystem2/Action
  If1/3 -> If Action Subsystem1/Action
  Merge1/1 -> Angle_output/1
  If Action Subsystem1/1(Out1) -> Merge1/3
  If Action Subsystem2/1(Out1) -> Merge1/1
  Angle_input/1 -> If Action Subsystem3/1(In1), If Action Subsystem1/1(In1), If Action Subsystem2/1(In1), If1/1
  If Action Subsystem3/1(Out1) -> Merge1/2

== system Flux_Nonsensor_pmsm/FOC电机控制/Flux_Observer/Flux_OBSERVER/PLL/integrator/Angle_Limit/If Action Subsystem1 ==
  In1 : Inport
  Action Port : ActionPort  ActionPortLabel=else
  Out1 : Outport
  wires:
  In1/1 -> Out1/1

== system Flux_Nonsensor_pmsm/FOC电机控制/Flux_Observer/Flux_OBSERVER/PLL/integrator/Angle_Limit/If Action Subsystem2 ==
  In1 : Inport
  Action Port : ActionPort  ActionPortLabel=if(u1 > 6.283185307)
  2pi : Constant  Value=2*pi  OutDataTypeStr=single
  Subtract1 : Sum  Inputs=+-  OutDataTypeStr=single
  Out1 : Outport
  wires:
  In1/1 -> Subtract1/1
  Subtract1/1 -> Out1/1
  2pi/1 -> Subtract1/2

== system Flux_Nonsensor_pmsm/FOC电机控制/Flux_Observer/Flux_OBSERVER/PLL/integrator/Angle_Limit/If Action Subsystem3 ==
  In1 : Inport
  Action Port : ActionPort  ActionPortLabel=elseif(u1<0)
  Angle_offset : Constant  Value=2*pi  OutDataTypeStr=single
  Subtract1 : Sum
  Out1 : Outport
  wires:
  In1/1 -> Subtract1/1
  Subtract1/1 -> Out1/1
  Angle_offset/1 -> Subtract1/2
